simulink library "Hot_Water_Datafile"  (R2018b)
settings: Solver=ode45  StartTime=0.0  StopTime=10.0  RelTol=1e-3  EnableMultiTasking=on
undefined symbols (not defined in the file): path_carnot
libraries: carnot x6
settings Model: Creator=lena.frank  LastModifiedBy=P41573
settings DataIOCC: LimitDataPoints=on  SaveFormat=Array  SignalLoggingSaveFormat=ModelDataLogs
settings OptimizationCC: ExpressionDepthLimit=2147483647  LifeSpan=inf
settings DebuggingCC: UnderspecifiedInitializationDetection=Classic  MergeDetectMultiDrivingBlocksExec=none  SolverPrmCheckMsg=warning  FcnCallInpInsideContextMsg=warning  StateNameClashWarn=warning  SFUnexpectedBacktrackingDiag=warning  SFNoUnconditionalDefaultTransitionDiag=warning  SFExecutionAtInitializationDiag=none
settings HardwareCC: ProdBitPerPointer=32  ProdBitPerSizeT=32  ProdBitPerPtrDiffT=32  ProdLargestAtomicFloat=None  ProdIntDivRoundTo=Undefined  ProdEndianess=Unspecified  ProdWordSize=32  ProdHWDeviceType=32-bit Generic
settings ModelReferenceCC: PropagateSignalLabelsOutOfModel=off
settings SFSimCC: SimUseLocalCustomCode=off
settings RTWCC: RTWUseLocalCustomCode=off
settings CodeAppCC: StateflowObjectComments=on
settings GRTTargetCC: TargetLangStandard=C89/C90 (ANSI)  GeneratePreprocessorConditionals=Disable all  CombineOutputUpdateFcns=off  GRTInterface=on
settings ConfigComp: CovMetricSettings=dw  CovHtmlReporting=on  CovSaveCumulativeToWorkspaceVar=on  CovSaveSingleToWorkspaceVar=on  CovExternalEMLEnable=off

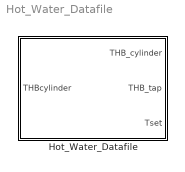
== system Hot_Water_Datafile ==
  Hot_Water_Datafile : Subsystem  mask(Hot Water Datafile){PathName=path_carnot('data'), FileName='DHWcalc_SFH_200L.mat', Thot=45, Tcold=10, Tamp=3, dshift=-137}
      mask prompts: PathName "Path"; FileName "File"; Thot "Tapping temperature setpoint in °C"; Tcold "Mean temperature in °C"; Tamp "Amplitude of the sine in K"; dshift "Phase shift of the sine in [days]"
      mask help:
      | Hot water consumption with a temperature and massflow profile from a file.
      | The file must contain a matrix with
      | column 1 : time in s
      | column 2 : temperature setpoint for hot water draw-offs in °C
      | Files max be created with the DHW-calc software and the scrpit createDatafile.m.
      | The hot water of the cylinder entering the block is mixed with the cold water to reach the temperature setpoint. The necessary massflow through the cylinder is calculated by this block and set in the outport to the cylinder.
      mask init:
      | [ok,VariableName] = CarnotCallbacks_Data_from_File('LoadData', ...
      |     gcbh, PathName, FileName);
      mask Help: web(fullfile(path_carnot('help'),'HotWaterDatafile.html'),'-helpbrowser')
      mask TypeOptions PathName: Data_from_File/PathName
      mask TypeOptions FileName: Data_from_File/FileName
      mask TypeOptions Thot: T_hot_water/Value
      mask TypeOptions Tcold: T_cold_Water_Sine/T
      mask TypeOptions Tamp: T_cold_Water_Sine/Tamp
      mask TypeOptions dshift: T_cold_Water_Sine/dshift
      mask DialogControl Container4 Prompt: Datafile
      mask DialogControl Control2 Prompt: From selected path
      mask DialogControl Control2 Callback: ok = CarnotCallbacks_Data_from_File('GetFilename',gcbh, 'selected');
      mask DialogControl Control3 Prompt: Carnot public data
      mask DialogControl Control3 Callback: ok = CarnotCallbacks_Data_from_File('GetFilename',gcbh, 'public');
      mask DialogControl Control4 Prompt: Carnot internal data
      mask DialogControl Control4 Callback: ok = CarnotCallbacks_Data_from_File('GetFilename',gcbh, 'internal');
      mask DialogControl Container3 Prompt: Cold water parameters
      mask Display:
      | text(15,120,'T-Mdot-Profile')
      | plot(0,0,140,130,[70,76,78,63,65,70,70,10],[80,78,74,74,78,80,100,100],[23,23,20,10],[43,47,50,50],[10,10,20,28,30,10],[30,20,20,23,30,30],[22,17],[54,54],[20,20],[54,50],[90,90,50,50],[10,-0,-0,10],[63,64],[60,72],[61,62],[38,50],[60,61],[13,27],[90,85,81,76,70,65,59,54,50],[6,4,6,4,6,4,5,3,5],[68,69],[56,68],[68,68],[32,44],[67,67],[13,23],[73,73],[61,71],[73,73],[43,52],[74,73],[21,36],[78,77],[56,67],[79,79],[34,45],[78,77],[9,23],[82,81],[14,26])

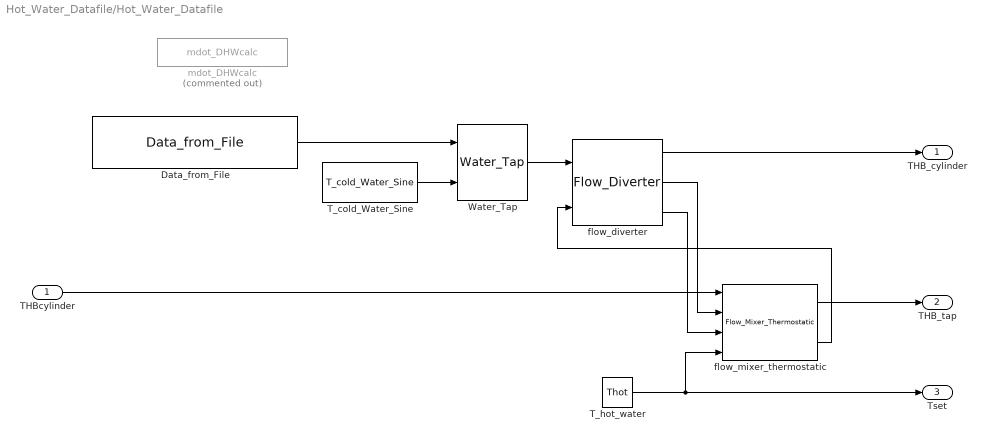
== system Hot_Water_Datafile/Hot_Water_Datafile ==
  THBcylinder : Inport
  Data_from_File : carnot/Load/General/Data_from_File  PathName=PathName  FileName=FileName  UserParam=off  DataName=DataName  t_sample=60
      settings: SourceProductName=Carnot
  T_cold_Water_Sine : carnot/Load/Hot_Water_Tapping/T_cold_Water_Sine  T=Tcold  Tamp=Tamp  dshift=dshift
      settings: SourceProductName=Carnot
  T_hot_water : Constant  Value=Thot
  Water_Tap : carnot/Load/Hot_Water_Tapping/Water_Tap  dia=0.02  p=2e5
      settings: SourceProductName=Carnot
  flow_diverter : carnot/Hydraulics/Flow_Diverter
      settings: SourceProductName=Carnot
  flow_mixer_thermostatic : carnot/Hydraulics/Flow_Mixer_Thermostatic  t=10
      settings: SourceProductName=Carnot
  mdot_DHWcalc : carnot/Load/Hot_Water_Tapping/mdot_DHWcalc  Commented=on  file=SFH_4P_200L_DHW  ext=.mat  dt=60
      settings: SourceProductName=Carnot
  THB_cylinder : Outport
  THB_tap : Outport  Port=2
  Tset : Outport  Port=3
  wires:
  flow_diverter/3 -> flow_mixer_thermostatic/3
  flow_diverter/2 -> flow_mixer_thermostatic/2
  flow_diverter/1 -> THB_cylinder/1
  THBcylinder/1 -> flow_mixer_thermostatic/1
  flow_mixer_thermostatic/1 -> THB_tap/1
  flow_mixer_thermostatic/2 -> flow_diverter/2
  Water_Tap/1 -> flow_diverter/1
  T_hot_water/1 -> flow_mixer_thermostatic/4, Tset/1
  T_cold_Water_Sine/1 -> Water_Tap/2
  Data_from_File/1 -> Water_Tap/1
